simulink model "impedanceControlNewWBI"  (R2014b)
settings: Solver=FixedStepDiscrete  StartTime=0.0  StopTime=10  FixedStep=Ts  RelTol=1e-3
InitFcn:
  | init;
libraries: WBCLibrary x3
settings Model: Creator=daniele  LastModifiedBy=pucci

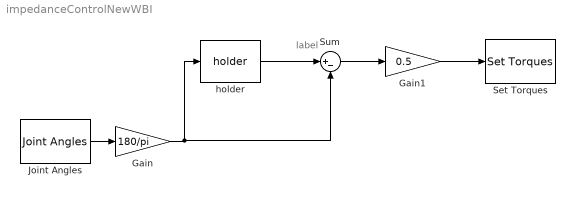
== system impedanceControlNewWBI ==
  note: label
  Gain : Gain  Gain=180/pi
  Gain1 : Gain  Gain=0.5
  Joint Angles : WBCLibrary/wholeBodyStates/Joint Angles  robotName=robotName  localName=localName
  Set Torques : WBCLibrary/wholeBodyActuators/Set Torques  val=6  robotName=robotName  localName=localName
  Sum : Sum  Inputs=|+-
  "holder " : WBCLibrary/Utilities/holder 
  wires:
  Joint Angles/1 -> Gain/1
  Gain/1 -> Sum/2, "holder "/1
  "holder "/1 -> Sum/1
  Sum/1 -> Gain1/1
  Gain1/1 -> Set Torques/1
